simulink model "hip_controller_2026_01_27"  (R2024b)
settings: Solver=FixedStepAuto  StartTime=0.0  StopTime=simDuration  FixedStep=0.01  RelTol=1e-3  EnableMultiTasking=on
InitFcn:
  | breakp=[-1, -0.8, -0.6, -0.4, -0.2, -0.1, 0, 0.1, 0.2, 0.4, 0.6, 0.8, 1];
  | splinenew =[-1, -0.8, -0.6, -0.4, -0.2, -0.1, 0, 0, 0.005, 0.01, 0.015,0.02,0.025];
undefined symbols (not defined in the file or in its folder): Discrete, K, qbreak, Time
libraries: simulink x53, arduinolib x11, dspswit3 x9, ctrlSharedLib x2, dspfdesign x2, slpidlib x2
(part 1 of 4)
settings Model: ExtModeTrigDuration=2  Creator=Aries  LastModifiedBy=zglin
settings SolverCC: ConcurrentTasks=on  AlgebraicLoopSolver=TrustRegion  PositivePriorityOrder=on  AutoInsertRateTranBlk=on
settings DataIOCC: SaveFormat=Array  ReturnWorkspaceOutputs=off
settings OptimizationCC: ReuseModelBlockBuffer=off  PassReuseOutputArgsAs=Individual arguments  MaxStackSize=64  EfficientTunableParamExpr=on
settings DebuggingCC: ParameterTunabilityLossMsg=error  UnconnectedInputMsg=warning  UnconnectedOutputMsg=warning  UnconnectedLineMsg=warning  ArithmeticOperatorsInVariantConditions=warning
settings HardwareCC: ProdBitPerPointer=32  ProdBitPerSizeT=32  ProdBitPerPtrDiffT=32  ProdLargestAtomicInteger=Long  ProdLargestAtomicFloat=Double  ProdWordSize=32  ProdHWDeviceType=ARM Compatible->ARM Cortex
settings ModelReferenceCC: EnableRefExpFcnMdlSchedulingChecks=on
settings SFSimCC: SimUseLocalCustomCode=off  MATLABDynamicMemAlloc=off  CustomCodeUndefinedFunction=UseInterfaceOnly
settings RTWCC: Description=Embedded Coder  SystemTargetFile=ert.tlc  HardwareBoard=Arduino MKR WiFi 1010  TemplateMakefile=ert_default_tmf  GenerateReport=on  RTWUseLocalCustomCode=off  Toolchain=Arduino ARM  BuildConfiguration=Faster Runs  LaunchReport=on  GPUComputeCapability=3.5  DLArmComputeVersion=19.05
settings CodeAppCC: ForceParamTrailComments=on  IgnoreCustomStorageClasses=off  OperatorAnnotations=on  StateflowObjectComments=on  MATLABSourceComments=on
settings ERTTargetCC: SupportContinuousTime=on  SupportNonInlinedSFcns=on  SupportVariableSizeSignals=on  ExtModeTransport=3  ExtModeStaticAlloc=on  ExtModeStaticAllocSize=8192  ExtModeMexFile=ext_xcp  ExtModeIntrfLevel=Level2 - Open  InlinedParameterPlacement=Hierarchical  DynamicArrayContainerType=coder::array
settings ConfigComp: CovMetricSettings=dswe

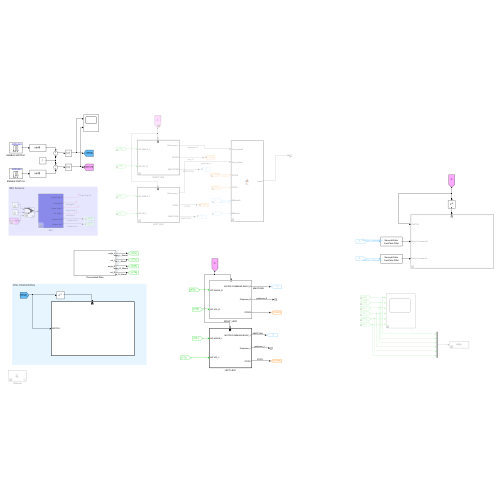
[thumbnail: Simulink's stored preview of the top-level diagram]
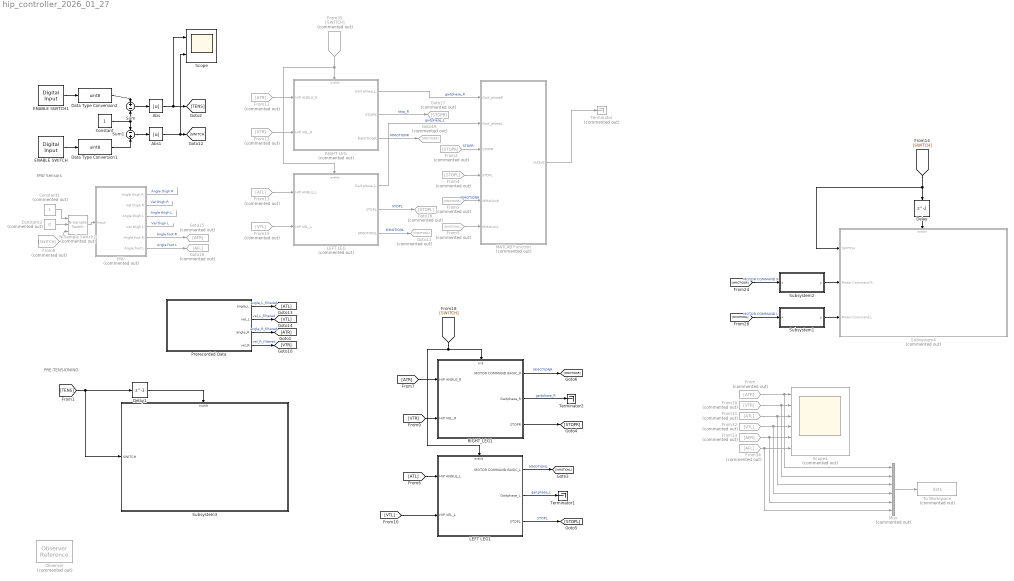
== system hip_controller_2026_01_27 ==
  note: IMU Sensors
  note: PRE-TENSIONING
  Abs : Abs  SaturateOnIntegerOverflow=off
  Abs1 : Abs  SaturateOnIntegerOverflow=off
  Constant : Constant
  Constant1 : Constant  Commented=on
  Constant3 : Constant  Commented=on  Value=0
  Data Type Conversion1 : DataTypeConversion  OutDataTypeStr=uint8  SaturateOnIntegerOverflow=off  RndMeth=Floor
  Data Type Conversion2 : DataTypeConversion  OutDataTypeStr=uint8  SaturateOnIntegerOverflow=off  RndMeth=Floor
  Delay : Delay
  Delay1 : Delay  DelayLength=1
  ENABLE SWITCH : arduinolib/Digital Input  pinNumber=6  mode=Input Pullup  Direction=input  SampleTime=0.01  blockPlatform=arduino
      settings: SourceProductName=Common
  ENABLE SWITCH1 : arduinolib/Digital Input  pinNumber=4  mode=Input Pullup  Direction=input  SampleTime=0.01  blockPlatform=arduino
      settings: SourceProductName=Common
  From : From  Commented=on  GotoTag=ATR
  From11 : From  Commented=on  GotoTag=ATR
  From12 : From  Commented=on  GotoTag=VTR
  From13 : From  Commented=on  GotoTag=ATL
  From15 : From  Commented=on  GotoTag=VTL
  From2 : From  Commented=on  GotoTag=STOPR
  From3 : From  Commented=on  GotoTag=MMOTIONR
  From30 : From  Commented=on  GotoTag=VTR
  From31 : From  Commented=on  GotoTag=ATL
  From32 : From  Commented=on  GotoTag=VTL
  From33 : From  Commented=on  GotoTag=AFR
  From34 : From  Commented=on  GotoTag=AFL
  From35 : From  Commented=on  GotoTag=SWITCH
  From4 : From  Commented=on  GotoTag=STOPL
  From5 : From  Commented=on  GotoTag=MMOTIONL
  From8 : From  Commented=on  GotoTag=SWITCH
  Goto11 : Goto  Commented=on  GotoTag=MMOTIONL
  Goto15 : Goto  Commented=on  GotoTag=AFR
  Goto16 : Goto  Commented=on  GotoTag=AFL
  Goto17 : Goto  Commented=on  GotoTag=STOPR
  Goto18 : Goto  Commented=on  GotoTag=STOPL
  Goto19 : Goto  Commented=on  GotoTag=MMOTIONR
  IMU : Subsystem  Commented=on
  LEFT LEG : Subsystem  Commented=on
  LEFT LEG1 : Subsystem
  MATLAB Function : MATLAB Function  Commented=on  TreatAsAtomicUnit=on
  Mux : Mux  Commented=on  Inputs=6
  N-Sample Switch2 : dspswit3/N-Sample Switch  Commented=on  N=10  reset=on  TriggerType=Rising edge  Ts=-1
  Observer : ObserverReference  Commented=on  ObserverModelName=hip_controller_181225_Observer1
  Prerecorded Data : Subsystem
  RIGHT LEG : Subsystem  Commented=on
  RIGHT_LEG1 : Subsystem
      settings: PortSchema="{\"entries\":[{\"content\":{\"sides\":[{\"content\":{\"connectorIds\":[\"In1\",\"In2\"]},\"type\":\"ConnectorPlacement.EquallySpacedRectSide\",\"uuid\":\"3c7f0152-c48a-47e5-a5d6-06ce9a094da4\"},{\"content\":{\"connectorIds\":[\"Out1\",\"Out2\",\"Out3\"],\"side\":\"RIGHT\"},\"type\":\"ConnectorPlacement.EquallySpacedRectSide\",\"uuid\":\"7e131d28-dc3d-49bf-b06d-5233735629db\"},{\"content\":{\"connectorIds\":[\"In3\"],\"side\":\"TOP\"},\"type\":\"ConnectorPlacement.EquallySpacedRectSide\",\"uuid\":\"34b65df0-5bb0-4402-bac3-467a5037582a\"}]},\"type\":\"ConnectorPlacement.EquallySpacedConnector\",\"uuid\":\"f00ff79e-fc41-40e3-bf13-a356f406cdad\"}],\"packageUris\":[\"http://schema.mathworks.com/mf0/Connector/R2020b\"],\"version\":\"1.0\"}"
  Scope : Scope  NumInputPorts=2
  Scope1 : Scope  Commented=on  NumInputPorts=6
  Subsystem1 : Subsystem  mask{wn=60, zt=1, x0=0}
      mask prompts: wn "Cut-off frequency (rad/s)"; zt "Damping ratio"; x0 "Initial Condition"
      mask Display: disp('Second-Order\nLow-Pass Filter');
  Subsystem2 : Subsystem  mask{wn=60, zt=1, x0=0}
      mask prompts: wn "Cut-off frequency (rad/s)"; zt "Damping ratio"; x0 "Initial Condition"
      mask Display: disp('Second-Order\nLow-Pass Filter');
  Subsystem3 : Subsystem
  Subsystem4 : Subsystem  Commented=on
  Sum : Sum  Inputs=+-
  Sum1 : Sum  Inputs=-+
  Terminator : Terminator  Commented=on
  Terminator1 : Terminator
  Terminator2 : Terminator
  To Workspace : ToWorkspace  Commented=on  VariableName=data  SampleTime=-1
      settings: Save2DSignal=2-D array (concatenate along first dimension)
  wires:
  [SWITCH] -> Delay/1, Subsystem4/1(SWITCH)
  Delay/1 -> Subsystem4/Enable
  From31/1 -> Scope1/3, Mux/3
  Constant3/1 -> N-Sample Switch2/2
  [MMOTIONL] -> Subsystem1/1(x)  "MOTOR COMMAND L"
  From34/1 -> Scope1/6, Mux/6
  From8/1 -> N-Sample Switch2/3
  From33/1 -> Scope1/5, Mux/5
  [MMOTIONR] -> Subsystem2/1(x)  "MOTOR COMMAND R"
  LEFT LEG/3(MMOTIONL) -> Goto11/1  "MMOTIONL"
  Constant1/1 -> N-Sample Switch2/1
  IMU/6(Angle foot L) -> Goto16/1  "Angle foot L"
  From13/1 -> LEFT LEG/1(HIP ANGLE_L)
  RIGHT LEG/2(STOPR) -> Goto17/1  "stop_R"
  Mux/1 -> To Workspace/1
  From12/1 -> RIGHT LEG/2(HIP VEL_R)
  N-Sample Switch2/1 -> IMU/1(Input)
  ENABLE SWITCH/1 -> Data Type Conversion1/1
  From35/1 -> RIGHT LEG/Enable, LEFT LEG/Enable
  Data Type Conversion1/1 -> Sum1/2
  RIGHT LEG/3(MMOTIONR) -> Goto19/1  "MMOTIONR"
  From11/1 -> RIGHT LEG/1(HIP ANGLE_R)
  IMU/1(Angle thigh R) -> ?  "Angle thigh R"
  From30/1 -> Mux/2, Scope1/2
  IMU/2(Vel thigh R) -> ?  "Vel thigh R"
  From32/1 -> Scope1/4, Mux/4
  IMU/5(Angle foot R) -> Goto15/1  "Angle foot R"
  From/1 -> Mux/1, Scope1/1
  IMU/4(Vel thigh L) -> ?  "Vel thigh L"
  IMU/3(Angle thigh L) -> ?  "Angle thigh L"
  LEFT LEG/2(STOPL) -> Goto18/1  "STOPL"
  From15/1 -> LEFT LEG/2(HIP VEL_L)
  Subsystem2/1(y) -> Subsystem4/2(Motor Command R)
  Subsystem1/1(y) -> Subsystem4/3(Motor Command L)
  ENABLE SWITCH1/1 -> Data Type Conversion2/1
  Data Type Conversion2/1 -> Sum/1
  Constant/1 -> Sum/2, Sum1/1
  Sum1/1 -> Abs1/1
  Sum/1 -> Abs/1
  Abs/1 -> Scope/1, [TENS]
  Abs1/1 -> Scope/2, [SWITCH]
  Delay1/1 -> Subsystem3/Enable
  [TENS] -> Subsystem3/1(SWITCH), Delay1/1
  RIGHT LEG/1(Gait phase_L) -> MATLAB Function/1(Gait_phaseR)  "gaitphase_R"
  LEFT LEG/1(Gait phase_L) -> MATLAB Function/2(Gait_phaseL)  "gaitphase_L"
  Prerecorded Data/1(angle_L) -> [ATL]  "angle_L_filtered"
  Prerecorded Data/2(vel_L) -> [VTL]  "vel_L_filtered"
  Prerecorded Data/3(angle_R) -> [ATR]  "angle_R_filtered"
  Prerecorded Data/4(vel_R) -> [VTR]  "vel_R_filtered"
  From2/1 -> MATLAB Function/3(STOPR)  "STOPR"
  From3/1 -> MATLAB Function/5(MMotionR)  "MMOTIONR"
  From4/1 -> MATLAB Function/4(STOPL)
  From5/1 -> MATLAB Function/6(MMotionL)
  MATLAB Function/1(output) -> Terminator/1
  RIGHT_LEG1/1(MOTOR COMMAND BASIC_R) -> [MMOTIONR]  "MMOTIONR"
  [VTL] -> LEFT LEG1/2(HIP VEL_L)
  [ATL] -> LEFT LEG1/1(HIP ANGLE_L)
  LEFT LEG1/3(STOPL) -> [STOPL]  "STOPL"
  [VTR] -> RIGHT_LEG1/2(HIP VEL_R)
  [SWITCH] -> RIGHT_LEG1/3(In3), LEFT LEG1/Enable
  LEFT LEG1/2(Gaitphase_L) -> Terminator1/1  "gaitphase_L"
  [ATR] -> RIGHT_LEG1/1(HIP ANGLE_R)
  LEFT LEG1/1(MOTOR COMMAND BASIC_L) -> [MMOTIONL]  "MMOTIONL"
  RIGHT_LEG1/3(STOPR) -> [STOPR]
  RIGHT_LEG1/2(Gaitphase_R) -> Terminator2/1  "gaitphase_R"

== system hip_controller_2026_01_27/IMU ==
  Input : Inport
  Data Type Conversion2 : DataTypeConversion  OutDataTypeStr=double  SaturateOnIntegerOverflow=off  RndMeth=Floor
  Demux : Demux  Outputs=6
  Gain{,2,4..5} (4 alike) : Gain  Gain=-pi/180
  Gain1 : Gain  Gain=pi/180
  Gain3 : Gain  Gain=pi/180
  IMUs (2 Thighs + 2 Feet) : arduinolib/I2C Read  I2CModule=0  Mode=Master  SlaveAddress=45  SlaveByteOrder=LittleEndian  Direction=Receiver  RegisterAddressMode=off  RegisterAddress=0  SlaveDataType=single  DataLength=6  NoAck=off  RepeatedStart=off  OutputStatus=off  blockPlatform=ARDUINO  SampleTime=0.01
      settings: SourceProductName=Common
  Remove offset : Subsystem
  Sum : Sum  Inputs=+-
  Angle thigh R : Outport
  Vel thigh R : Outport  Port=2
  Angle thigh L : Outport  Port=3
  Vel thigh L : Outport  Port=4
  Angle foot R : Outport  Port=5
  Angle foot L : Outport  Port=6
  wires:
  IMUs (2 Thighs + 2 Feet)/1 -> Data Type Conversion2/1
  Demux/5 -> Gain4/1  "Angle foot R"
  Demux/4 -> Gain3/1  "Vel thigh L"
  Demux/3 -> Gain/1  "Angle thigh L"
  Demux/2 -> Gain2/1  "Vel thigh R"
  Demux/1 -> Gain1/1  "Angle thigh R"
  Demux/6 -> Gain5/1  "Angle foot L"
  Input/1 -> Remove offset/Enable
  Data Type Conversion2/1 -> Sum/1, Remove offset/1(Input)
  Sum/1 -> Demux/1
  Remove offset/1(Mean value) -> Sum/2
  Gain/1 -> Angle thigh L/1
  Gain1/1 -> Angle thigh R/1
  Gain2/1 -> Vel thigh R/1
  Gain3/1 -> Vel thigh L/1
  Gain4/1 -> Angle foot R/1
  Gain5/1 -> Angle foot L/1

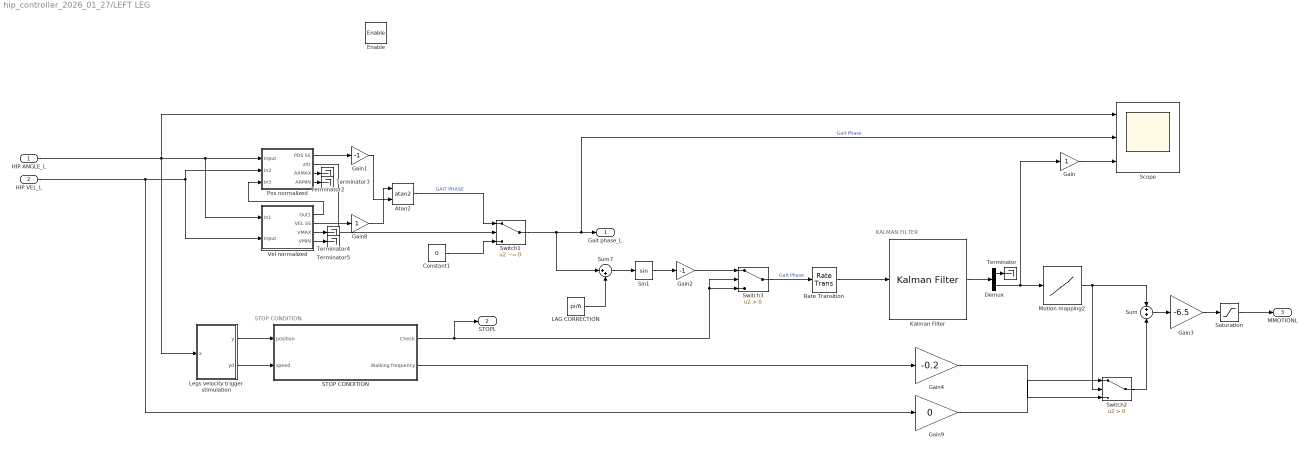
== system hip_controller_2026_01_27/LEFT LEG ==
  note: STOP CONDITION
  note: KALMAN FILTER
  HIP ANGLE_L : Inport
  HIP VEL_L : Inport  Port=2
  Enable : EnablePort  StatesWhenEnabling=reset
  Atan2 : Trigonometry  Operator=atan2
  Constant1 : Constant  Value=0
  Demux : Demux  Outputs=2
  Gain : Gain
  Gain1 : Gain  Gain=-1
  Gain2 : Gain  Gain=-1
  Gain3 : Gain  Gain=-6.5
  Gain4 : Gain  Gain=-0.2
  Gain8 : Gain
  Gain9 : Gain  Gain=0
  Kalman Filter : ctrlSharedLib/Kalman Filter  TimeDomain=Discrete-Time  UseCurrentEstimator=on  ModelSource=Individual A, B, C, D matrices  ModelSourceVariable=idss  A=[1 0.01;0 1]  B=eye(2)  C=[1 0]  D=zeros(2)  NumberOfStates=1  NumberOfInputs=1  NumberOfOutputs=1  InitialEstimateSource=Dialog  X0=0  P0=10  UseK=off  UseGH=off  NumberOfProcessNoiseInputs=2  G=1  TimeInvariantG=on  H=0  TimeInvariantH=on  Q=0.02  TimeInvariantQ=on  R=0.75  TimeInvariantR=on  N=0  TimeInvariantN=on  AddInputPort=off  AddEnablePort=off  OutputEstimatedY=off  OutputP=off  Ts=-1
  LAG CORRECTION : Constant  Value=pi/6
  Legs velocity trigger stimulation : Subsystem  mask{wn=10, zt=1, x0=0}
      mask prompts: wn "Cut-off frequency (rad/s)"; zt "Damping ratio"; x0 "Initial Condition"
      mask Display: disp('Second-Order\nLow-Pass Filter');
  Motion mapping2 : Lookup_n-D  NumberOfTableDimensions=1  BreakpointsForDimension1=breakp  BreakpointsForDimension2=qbreak(:,2)  Table=splinenew  InterpMethod=Cubic spline  ExtrapMethod=Cubic spline  InternalRulePriority=Speed  RndMeth=Simplest
  Pos normalized : Subsystem
  Rate Transition : RateTransition  OutPortSampleTime=0.01
  STOP CONDITION : Subsystem
  Saturation : Saturate  UpperLimit=600*pi/180  LowerLimit=-600*pi/180
  Scope : Scope  NumInputPorts=3
  Sin1 : Trigonometry
  Sum : Sum
  Sum7 : Sum  Inputs=|++
  Switch1 : Switch  Criteria=u2 ~= 0  SaturateOnIntegerOverflow=off  InputSameDT=off
  Switch2 : Switch  Criteria=u2 > Threshold  SaturateOnIntegerOverflow=off  InputSameDT=off
  Switch3 : Switch  Criteria=u2 > Threshold  SaturateOnIntegerOverflow=off  InputSameDT=off
  Terminator{,2..5} (5 alike) : Terminator
  Vel normalized : Subsystem
  Gait phase_L : Outport
  STOPL : Outport  Port=2
  MMOTIONL : Outport  Port=3
  wires:
  Kalman Filter/1 -> Demux/1
  Gain8/1 -> Atan2/1
  Gain2/1 -> Switch3/1
  STOP CONDITION/1(Check) -> STOPL/1, Switch3/2, Switch3/3
  Gain3/1 -> Saturation/1
  Rate Transition/1 -> Kalman Filter/1
  Atan2/1 -> Switch1/1  "GAIT PHASE"
  Sin1/1 -> Gain2/1
  Switch1/1 -> Sum7/1, Scope/2, Gait phase_L/1  "Gait Phase"
  HIP VEL_L/1 -> Vel normalized/2(Input), Pos normalized/2(In2), Gain9/1
  Switch3/1 -> Rate Transition/1  "Gait Phase"
  Constant1/1 -> Switch1/3
  Motion mapping2/1 -> Sum/1, Switch2/2
  Sum/1 -> Gain3/1
  Demux/1 -> Terminator/1
  LAG CORRECTION/1 -> Sum7/2
  Sum7/1 -> Sin1/1
  Demux/2 -> Gain/1, Motion mapping2/1
  Gain1/1 -> Atan2/2
  Gain9/1 -> Switch2/1
  Gain4/1 -> Switch2/3
  Switch2/1 -> Sum/2
  STOP CONDITION/2(Walking frequency) -> Gain4/1
  Saturation/1 -> MMOTIONL/1
  HIP ANGLE_L/1 -> Legs velocity trigger stimulation/1(x), Scope/1, Vel normalized/1(In1), Pos normalized/1(Input)
  Pos normalized/1(POS SS) -> Gain1/1
  Pos normalized/2(z(t)) -> Switch1/2
  Vel normalized/1(Out1) -> Pos normalized/3(In3)
  Vel normalized/2(VEL SS) -> Gain8/1
  Pos normalized/3(ARMAX) -> Terminator2/1
  Pos normalized/4(ARMIN) -> Terminator3/1
  Vel normalized/3(VMAX) -> Terminator4/1
  Vel normalized/4(VMIN) -> Terminator5/1
  Gain/1 -> Scope/3
  Legs velocity trigger stimulation/1(y) -> STOP CONDITION/1(position)
  Legs velocity trigger stimulation/2(yd) -> STOP CONDITION/2(speed)

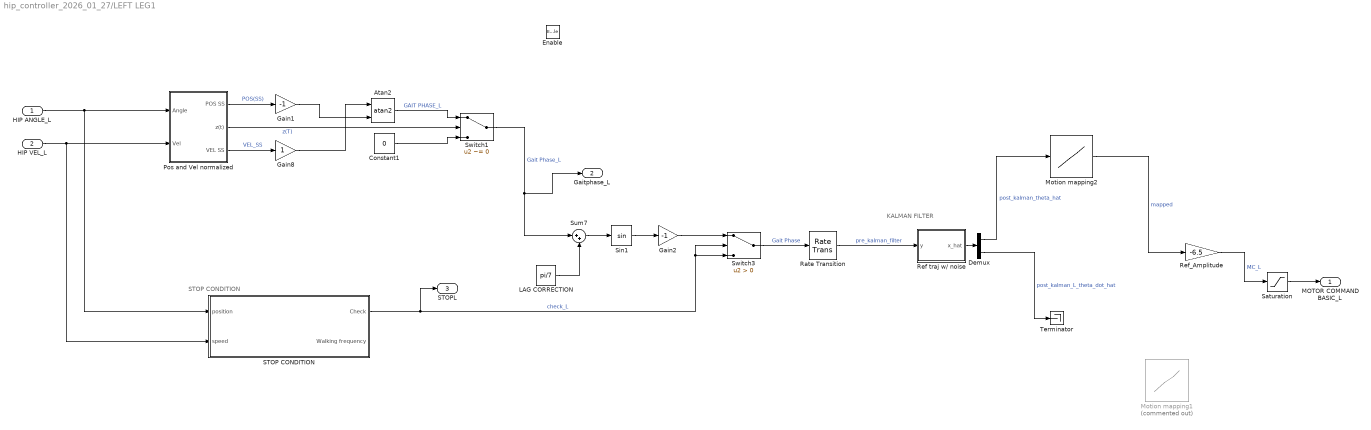
== system hip_controller_2026_01_27/LEFT LEG1 ==
  note: STOP CONDITION
  note: KALMAN FILTER
  HIP ANGLE_L : Inport
  HIP VEL_L : Inport  Port=2
  Enable : EnablePort
  Atan2 : Trigonometry  Operator=atan2
  Constant1 : Constant  Value=0
  Demux : Demux  Outputs=2
  Gain1 : Gain  Gain=-1
  Gain2 : Gain  Gain=-1
  Gain8 : Gain
  LAG CORRECTION : Constant  Value=pi/7
  Motion mapping1 : Lookup_n-D  Commented=on  NumberOfTableDimensions=1  BreakpointsForDimension1=[-1, -0.8, -0.6, -0.4, -0.2, -0.1, 0, 0.1, 0.2, 0.4, 0.6, 0.8, 1]  BreakpointsForDimension2=qbreak(:,2)  Table=[-1, -0.8, -0.6, -0.4, -0.2, -0.1, 0, 0, 0.005, 0.01, 0.015,0.02,0.025]  InterpMethod=Cubic spline  ExtrapMethod=Cubic spline  InternalRulePriority=Speed  RndMeth=Simplest
  Motion mapping2 : Lookup_n-D  NumberOfTableDimensions=1  BreakpointsForDimension1=breakp  BreakpointsForDimension2=qbreak(:,2)  Table=splinenew  InterpMethod=Cubic spline  ExtrapMethod=Cubic spline  InternalRulePriority=Speed  RndMeth=Simplest
  Pos and Vel normalized : Subsystem
  Rate Transition : RateTransition  OutPortSampleTime=0.01
  Ref traj w/ noise : MATLAB Function  TreatAsAtomicUnit=on
  Ref_Amplitude : Gain  Gain=-6.5
  STOP CONDITION : Subsystem
  Saturation : Saturate  UpperLimit=600*pi/180  LowerLimit=-600*pi/180
  Sin1 : Trigonometry
  Sum7 : Sum  Inputs=|++
  Switch1 : Switch  Criteria=u2 ~= 0  SaturateOnIntegerOverflow=off  InputSameDT=off
  Switch3 : Switch  Criteria=u2 > Threshold  SaturateOnIntegerOverflow=off  InputSameDT=off
  Terminator : Terminator
  MOTOR COMMAND BASIC_L : Outport
  Gaitphase_L : Outport  Port=2
  STOPL : Outport  Port=3
  wires:
  Gain8/1 -> Atan2/1
  Gain2/1 -> Switch3/1
  STOP CONDITION/1(Check) -> STOPL/1, Switch3/2, Switch3/3  "check_L"
  Atan2/1 -> Switch1/1  "GAIT PHASE_L"
  Sin1/1 -> Gain2/1
  Switch1/1 -> Sum7/1, Gaitphase_L/1  "Gait Phase_L"
  Switch3/1 -> Rate Transition/1  "Gait Phase"
  Constant1/1 -> Switch1/3
  LAG CORRECTION/1 -> Sum7/2
  Sum7/1 -> Sin1/1
  Gain1/1 -> Atan2/2
  Pos and Vel normalized/1(POS SS) -> Gain1/1  "POS(SS)"
  Pos and Vel normalized/2(z(t)) -> Switch1/2  "z(T)"
  Pos and Vel normalized/3(VEL SS) -> Gain8/1  "VEL_SS"
  Demux/1 -> Motion mapping2/1  "post_kalman_theta_hat"
  Motion mapping2/1 -> Ref_Amplitude/1  "mapped"
  Ref_Amplitude/1 -> Saturation/1  "MC_L"
  HIP VEL_L/1 -> Pos and Vel normalized/2(Vel), STOP CONDITION/2(speed)
  HIP ANGLE_L/1 -> Pos and Vel normalized/1(Angle), STOP CONDITION/1(position)
  Rate Transition/1 -> Ref traj w/ noise/1(y)  "pre_kalman_filter"
  Ref traj w/ noise/1(x_hat) -> Demux/1
  Demux/2 -> Terminator/1  "post_kalman_L_theta_dot_hat"
  Saturation/1 -> MOTOR COMMAND BASIC_L/1

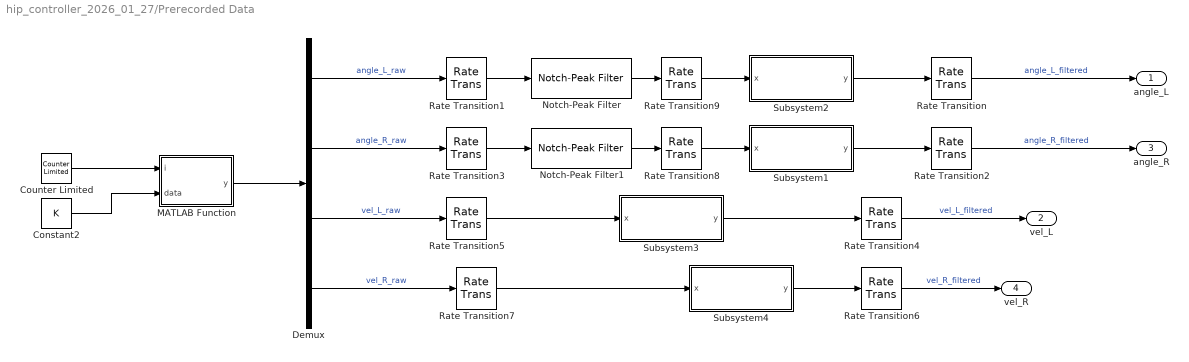
== system hip_controller_2026_01_27/Prerecorded Data ==
  Constant2 : Constant  Value=K
  Counter Limited : simulink/Sources/Counter Limited  uplimit=size(K,1)  tsamp=0.01
  Demux : Demux
  MATLAB Function : MATLAB Function  TreatAsAtomicUnit=on
  Notch-Peak Filter : dspfdesign/Notch-Peak Filter  Specification=Bandwidth and center frequency  BandwidthPort=off  Bandwidth=0.1  QualityFactorPort=off  QualityFactor=5  CenterFrequencyPort=off  CenterFrequency=0  BandwidthCoefficientPort=off  BandwidthCoefficient=0.72654  CenterFrequencyCoefficientPort=off  CenterFrequencyCoefficient=0  Output=Notch  SampleRateMode=Specify on dialog  SampleRate=100  SimulateUsing=Interpreted execution
  Notch-Peak Filter1 : dspfdesign/Notch-Peak Filter  Specification=Bandwidth and center frequency  BandwidthPort=off  Bandwidth=0.1  QualityFactorPort=off  QualityFactor=5  CenterFrequencyPort=off  CenterFrequency=0  BandwidthCoefficientPort=off  BandwidthCoefficient=0.72654  CenterFrequencyCoefficientPort=off  CenterFrequencyCoefficient=0  Output=Notch  SampleRateMode=Specify on dialog  SampleRate=100  SimulateUsing=Interpreted execution
  Rate Transition{,1..9} (10 alike) : RateTransition  OutPortSampleTime=0.01
  Subsystem1 : Subsystem  mask{wn=20, zt=1, x0=0}
      mask prompts: wn "Cut-off frequency (rad/s)"; zt "Damping ratio"; x0 "Initial Condition"
      mask Display: disp('Second-Order\nLow-Pass Filter');
  Subsystem2 : Subsystem  mask{wn=20, zt=1, x0=0}
      mask prompts: wn "Cut-off frequency (rad/s)"; zt "Damping ratio"; x0 "Initial Condition"
      mask Display: disp('Second-Order\nLow-Pass Filter');
  Subsystem3 : Subsystem  mask{wn=20, zt=1, x0=0}
      mask prompts: wn "Cut-off frequency (rad/s)"; zt "Damping ratio"; x0 "Initial Condition"
      mask Display: disp('Second-Order\nLow-Pass Filter');
  Subsystem4 : Subsystem  mask{wn=20, zt=1, x0=0}
      mask prompts: wn "Cut-off frequency (rad/s)"; zt "Damping ratio"; x0 "Initial Condition"
      mask Display: disp('Second-Order\nLow-Pass Filter');
  angle_L : Outport
  vel_L : Outport  Port=2
  angle_R : Outport  Port=3
  vel_R : Outport  Port=4
  wires:
  Notch-Peak Filter/1 -> Rate Transition9/1
  Rate Transition1/1 -> Notch-Peak Filter/1
  Rate Transition3/1 -> Notch-Peak Filter1/1
  MATLAB Function/1(y) -> Demux/1
  Counter Limited/1 -> MATLAB Function/1(i)
  Constant2/1 -> MATLAB Function/2(data)
  Notch-Peak Filter1/1 -> Rate Transition8/1
  Demux/1 -> Rate Transition1/1  "angle_L_raw"
  Demux/2 -> Rate Transition3/1  "angle_R_raw"
  Rate Transition2/1 -> angle_R/1  "angle_R_filtered"
  Rate Transition/1 -> angle_L/1  "angle_L_filtered"
  Subsystem2/1(y) -> Rate Transition/1
  Subsystem1/1(y) -> Rate Transition2/1
  Subsystem3/1(y) -> Rate Transition4/1
  Rate Transition5/1 -> Subsystem3/1(x)
  Rate Transition4/1 -> vel_L/1  "vel_L_filtered"
  Demux/3 -> Rate Transition5/1  "vel_L_raw"
  Rate Transition7/1 -> Subsystem4/1(x)
  Subsystem4/1(y) -> Rate Transition6/1
  Demux/4 -> Rate Transition7/1  "vel_R_raw"
  Rate Transition6/1 -> vel_R/1  "vel_R_filtered"
  Rate Transition9/1 -> Subsystem2/1(x)
  Rate Transition8/1 -> Subsystem1/1(x)

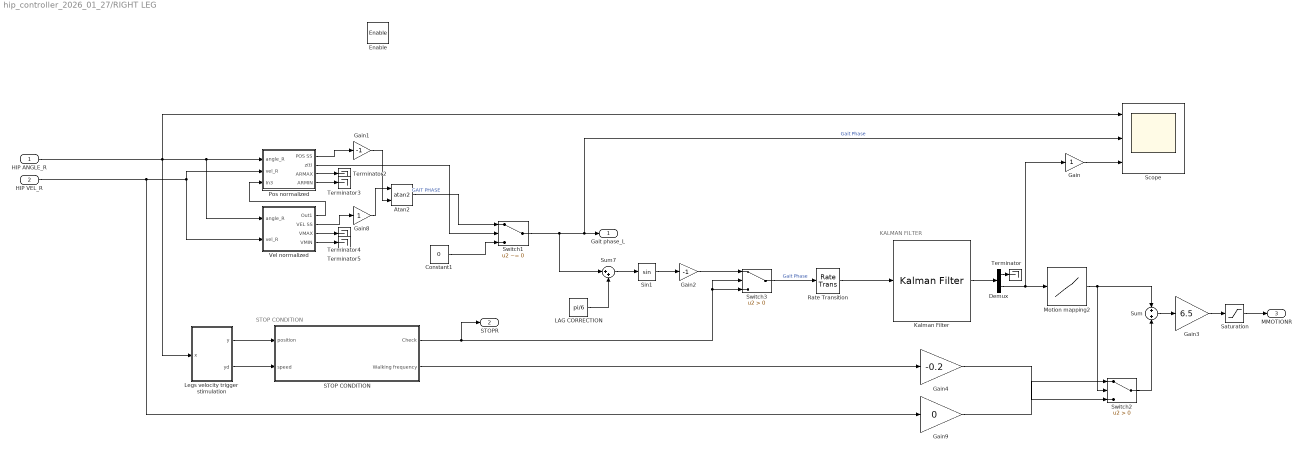
== system hip_controller_2026_01_27/RIGHT LEG ==
  note: STOP CONDITION
  note: KALMAN FILTER
  HIP ANGLE_R : Inport
  HIP VEL_R : Inport  Port=2
  Enable : EnablePort  StatesWhenEnabling=reset
  Atan2 : Trigonometry  Operator=atan2
  Constant1 : Constant  Value=0
  Demux : Demux  Outputs=2
  Gain : Gain
  Gain1 : Gain  Gain=-1
  Gain2 : Gain  Gain=-1
  Gain3 : Gain  Gain=6.5
  Gain4 : Gain  Gain=-0.2
  Gain8 : Gain
  Gain9 : Gain  Gain=0
  Kalman Filter : ctrlSharedLib/Kalman Filter  TimeDomain=Discrete-Time  UseCurrentEstimator=on  ModelSource=Individual A, B, C, D matrices  ModelSourceVariable=idss  A=[1 0.01;0 1]  B=eye(2)  C=[1 0]  D=zeros(2)  NumberOfStates=1  NumberOfInputs=1  NumberOfOutputs=1  InitialEstimateSource=Dialog  X0=0  P0=10  UseK=off  UseGH=off  NumberOfProcessNoiseInputs=2  G=1  TimeInvariantG=on  H=0  TimeInvariantH=on  Q=0.02  TimeInvariantQ=on  R=0.75  TimeInvariantR=on  N=0  TimeInvariantN=on  AddInputPort=off  AddEnablePort=off  OutputEstimatedY=off  OutputP=off  Ts=-1
  LAG CORRECTION : Constant  Value=pi/6
  Legs velocity trigger stimulation : Subsystem  mask{wn=10, zt=1, x0=0}
      mask prompts: wn "Cut-off frequency (rad/s)"; zt "Damping ratio"; x0 "Initial Condition"
      mask Display: disp('Second-Order\nLow-Pass Filter');
  Motion mapping2 : Lookup_n-D  NumberOfTableDimensions=1  BreakpointsForDimension1=breakp  BreakpointsForDimension2=qbreak(:,2)  Table=splinenew  InterpMethod=Cubic spline  ExtrapMethod=Cubic spline  InternalRulePriority=Speed  RndMeth=Simplest
  Pos normalized : Subsystem
  Rate Transition : RateTransition  OutPortSampleTime=0.01
  STOP CONDITION : Subsystem
  Saturation : Saturate  UpperLimit=600*pi/180  LowerLimit=-600*pi/180
  Scope : Scope  NumInputPorts=3
  Sin1 : Trigonometry
  Sum : Sum
  Sum7 : Sum  Inputs=|++
  Switch1 : Switch  Criteria=u2 ~= 0  SaturateOnIntegerOverflow=off  InputSameDT=off
  Switch2 : Switch  Criteria=u2 > Threshold  SaturateOnIntegerOverflow=off  InputSameDT=off
  Switch3 : Switch  Criteria=u2 > Threshold  SaturateOnIntegerOverflow=off  InputSameDT=off
  Terminator{,2..5} (5 alike) : Terminator
  Vel normalized : Subsystem
  Gait phase_L : Outport
  STOPR : Outport  Port=2
  MMOTIONR : Outport  Port=3
  wires:
  Kalman Filter/1 -> Demux/1
  Gain8/1 -> Atan2/1
  Gain2/1 -> Switch3/1
  STOP CONDITION/1(Check) -> STOPR/1, Switch3/2, Switch3/3
  Gain3/1 -> Saturation/1
  Rate Transition/1 -> Kalman Filter/1
  Atan2/1 -> Switch1/1  "GAIT PHASE"
  Sin1/1 -> Gain2/1
  Switch1/1 -> Sum7/1, Scope/2, Gait phase_L/1  "Gait Phase"
  HIP VEL_R/1 -> Vel normalized/2(vel_R), Pos normalized/2(vel_R), Gain9/1
  Switch3/1 -> Rate Transition/1  "Gait Phase"
  Constant1/1 -> Switch1/3
  Motion mapping2/1 -> Sum/1, Switch2/2
  Sum/1 -> Gain3/1
  Demux/1 -> Terminator/1
  LAG CORRECTION/1 -> Sum7/2
  Sum7/1 -> Sin1/1
  Demux/2 -> Gain/1, Motion mapping2/1
  Gain1/1 -> Atan2/2
  Gain9/1 -> Switch2/1
  Gain4/1 -> Switch2/3
  Switch2/1 -> Sum/2
  STOP CONDITION/2(Walking frequency) -> Gain4/1
  HIP ANGLE_R/1 -> Legs velocity trigger stimulation/1(x), Scope/1, Vel normalized/1(angle_R), Pos normalized/1(angle_R)
  Pos normalized/1(POS SS) -> Gain1/1
  Pos normalized/2(z(t)) -> Switch1/2
  Vel normalized/1(Out1) -> Pos normalized/3(In3)
  Vel normalized/2(VEL SS) -> Gain8/1
  Pos normalized/3(ARMAX) -> Terminator2/1
  Pos normalized/4(ARMIN) -> Terminator3/1
  Vel normalized/3(VMAX) -> Terminator4/1
  Vel normalized/4(VMIN) -> Terminator5/1
  Gain/1 -> Scope/3
  Legs velocity trigger stimulation/1(y) -> STOP CONDITION/1(position)
  Legs velocity trigger stimulation/2(yd) -> STOP CONDITION/2(speed)
  Saturation/1 -> MMOTIONR/1

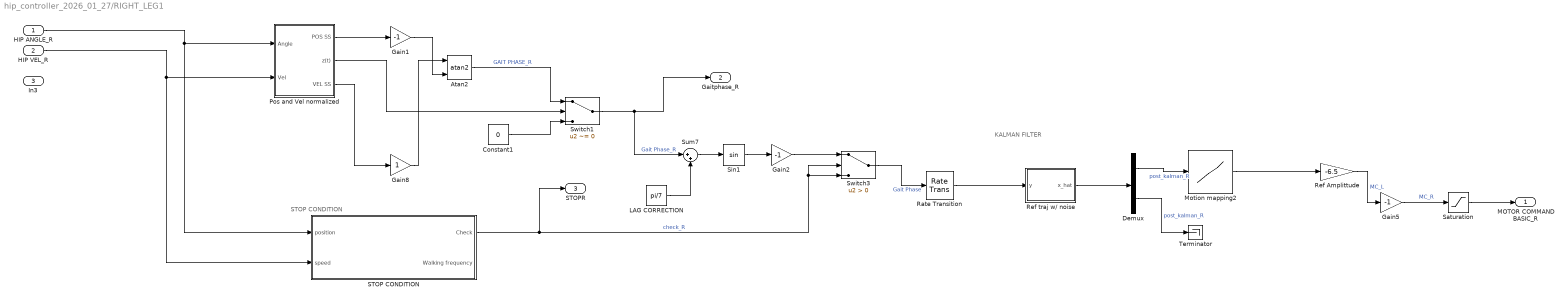
== system hip_controller_2026_01_27/RIGHT_LEG1 ==
  note: STOP CONDITION
  note: KALMAN FILTER
  HIP ANGLE_R : Inport
  HIP VEL_R : Inport  Port=2
  In3 : Inport  Port=3
  Atan2 : Trigonometry  Operator=atan2
  Constant1 : Constant  Value=0
  Demux : Demux  Outputs=2
  Gain1 : Gain  Gain=-1
  Gain2 : Gain  Gain=-1
  Gain5 : Gain  Gain=-1
  Gain8 : Gain
  LAG CORRECTION : Constant  Value=pi/7
  Motion mapping2 : Lookup_n-D  NumberOfTableDimensions=1  BreakpointsForDimension1=breakp  BreakpointsForDimension2=qbreak(:,2)  Table=splinenew  InterpMethod=Cubic spline  ExtrapMethod=Cubic spline  InternalRulePriority=Speed  RndMeth=Simplest
  Pos and Vel normalized : Subsystem
  Rate Transition : RateTransition  OutPortSampleTime=0.01
  Ref Amplittude : Gain  Gain=-6.5
  Ref traj w/ noise : MATLAB Function  TreatAsAtomicUnit=on
  STOP CONDITION : Subsystem
  Saturation : Saturate  UpperLimit=600*pi/180  LowerLimit=-600*pi/180
  Sin1 : Trigonometry
  Sum7 : Sum  Inputs=|++
  Switch1 : Switch  Criteria=u2 ~= 0  SaturateOnIntegerOverflow=off  InputSameDT=off
  Switch3 : Switch  Criteria=u2 > Threshold  SaturateOnIntegerOverflow=off  InputSameDT=off
  Terminator : Terminator
  MOTOR COMMAND BASIC_R : Outport
  Gaitphase_R : Outport  Port=2
  STOPR : Outport  Port=3
  wires:
  Gain8/1 -> Atan2/1
  Gain2/1 -> Switch3/1
  STOP CONDITION/1(Check) -> STOPR/1, Switch3/2, Switch3/3  "check_R"
  Atan2/1 -> Switch1/1  "GAIT PHASE_R"
  Sin1/1 -> Gain2/1
  Switch1/1 -> Sum7/1, Gaitphase_R/1  "Gait Phase_R"
  HIP VEL_R/1 -> Pos and Vel normalized/2(Vel), STOP CONDITION/2(speed)
  Switch3/1 -> Rate Transition/1  "Gait Phase"
  Constant1/1 -> Switch1/3
  LAG CORRECTION/1 -> Sum7/2
  Sum7/1 -> Sin1/1
  Gain1/1 -> Atan2/2
  Pos and Vel normalized/1(POS SS) -> Gain1/1
  Pos and Vel normalized/2(z(t)) -> Switch1/2
  Pos and Vel normalized/3(VEL SS) -> Gain8/1
  HIP ANGLE_R/1 -> STOP CONDITION/1(position), Pos and Vel normalized/1(Angle)
  Demux/1 -> Motion mapping2/1  "post_kalman_R"
  Motion mapping2/1 -> Ref Amplittude/1
  Gain5/1 -> Saturation/1  "MC_R"
  Ref Amplittude/1 -> Gain5/1  "MC_L"
  Rate Transition/1 -> Ref traj w/ noise/1(y)
  Ref traj w/ noise/1(x_hat) -> Demux/1
  Saturation/1 -> MOTOR COMMAND BASIC_R/1
  Demux/2 -> Terminator/1  "post_kalman_R"

== system hip_controller_2026_01_27/Subsystem1 ==
  x : Inport
  Constant : Constant  Value=2
  Integrator1 : Integrator  InitialConditionSource=external
  Integrator2 : Integrator
  Product : Product  RndMeth=Zero
  Product1 : Product  RndMeth=Zero
  Product2 : Product  Inputs=3  RndMeth=Zero
  Sum : Sum  Inputs=|+-
  Sum1 : Sum  Inputs=|+-
  wn : Constant  Value=wn
  x0 : Constant  Value=x0
  zt : Constant  Value=zt
  y : Outport  VectorParamsAs1DForOutWhenUnconnected=off
  wires:
  Sum/1 -> Product/2
  wn/1 -> Product/1, Product1/1
  Sum1/1 -> Sum/1
  x0/1 -> Integrator1/2
  Integrator2/1 -> Product1/2, Product2/1
  Product/1 -> Integrator2/1
  x/1 -> Sum1/1
  Product1/1 -> Integrator1/1
  Integrator1/1 -> Sum1/2, y/1
  Product2/1 -> Sum/2
  zt/1 -> Product2/3
  Constant/1 -> Product2/2

== system hip_controller_2026_01_27/Subsystem2 ==
  x : Inport
  Constant : Constant  Value=2
  Integrator1 : Integrator  InitialConditionSource=external
  Integrator2 : Integrator
  Product : Product  RndMeth=Zero
  Product1 : Product  RndMeth=Zero
  Product2 : Product  Inputs=3  RndMeth=Zero
  Sum : Sum  Inputs=|+-
  Sum1 : Sum  Inputs=|+-
  wn : Constant  Value=wn
  x0 : Constant  Value=x0
  zt : Constant  Value=zt
  y : Outport  VectorParamsAs1DForOutWhenUnconnected=off
  wires:
  Sum/1 -> Product/2
  wn/1 -> Product/1, Product1/1
  Sum1/1 -> Sum/1
  x0/1 -> Integrator1/2
  Integrator2/1 -> Product1/2, Product2/1
  Product/1 -> Integrator2/1
  x/1 -> Sum1/1
  Product1/1 -> Integrator1/1
  Integrator1/1 -> Sum1/2, y/1
  Product2/1 -> Sum/2
  zt/1 -> Product2/3
  Constant/1 -> Product2/2

== system hip_controller_2026_01_27/Subsystem3 ==
  note: RightLeg_AK60-6 Motor Modules
  note: LeftLeg_AK60-6 Motor Modules
  SWITCH : Inport
  Enable : EnablePort  StatesWhenEnabling=reset
  Abs : Abs  SaturateOnIntegerOverflow=off
  Abs1 : Abs  SaturateOnIntegerOverflow=off
  Chart : Stateflow chart  TreatAsAtomicUnit=on
  Chart1 : Stateflow chart  TreatAsAtomicUnit=on
  Data Type Conversion1 : DataTypeConversion  OutDataTypeStr=single  SaturateOnIntegerOverflow=off  RndMeth=Floor
  Data Type Conversion6 : DataTypeConversion  OutDataTypeStr=single  SaturateOnIntegerOverflow=off  RndMeth=Floor
  Left Motor Velocity : Subsystem
  Right Motor Velocity : Subsystem
  Subsystem1 : Subsystem  mask{wn=25, zt=1, x0=0}
      mask prompts: wn "Cut-off frequency (rad/s)"; zt "Damping ratio"; x0 "Initial Condition"
      mask Display: disp('Second-Order\nLow-Pass Filter');
  Subsystem4 : Subsystem  mask{wn=25, zt=1, x0=0}
      mask prompts: wn "Cut-off frequency (rad/s)"; zt "Damping ratio"; x0 "Initial Condition"
      mask Display: disp('Second-Order\nLow-Pass Filter');
  Terminator{1..6} (6 alike) : Terminator
  wires:
  Chart1/2(vel) -> Data Type Conversion1/1
  SWITCH/1 -> Chart1/2(ON_OFF), Chart/2(ON_OFF)
  Data Type Conversion6/1 -> Right Motor Velocity/2(Motor command)
  Left Motor Velocity/3(MOTOR TORQUE) -> Subsystem1/1(x)
  Right Motor Velocity/2(MOTOR SPEED) -> Terminator2/1
  Left Motor Velocity/2(MOTOR SPEED) -> Terminator1/1
  Chart/2(vel) -> Data Type Conversion6/1
  Right Motor Velocity/1(MOTOR POSITION) -> Terminator4/1
  Subsystem4/1(y) -> Abs/1  "TORQUE"
  Right Motor Velocity/3(MOTOR TORQUE) -> Subsystem4/1(x)
  Subsystem4/2(yd) -> Terminator5/1
  Abs/1 -> Chart/1(MOTOR_TORQUE)
  Left Motor Velocity/1(MOTOR POSITION) -> Terminator3/1
  Subsystem1/1(y) -> Abs1/1  "TORQUE"
  Subsystem1/2(yd) -> Terminator6/1
  Abs1/1 -> Chart1/1(MOTOR_TORQUE)
  Chart/1(enablestati) -> Right Motor Velocity/1(SWITCH)
  Chart1/1(enablestati) -> Left Motor Velocity/1(SWITCH)
  Data Type Conversion1/1 -> Left Motor Velocity/2(Motor command)

== system hip_controller_2026_01_27/Subsystem4 ==
  note: RightLeg_AK60-6 Motor Modules
  note: LeftLeg_AK60-6 Motor Modules
  SWITCH : Inport
  Motor Command R : Inport  Port=2
  Motor Command L : Inport  Port=3
  Enable : EnablePort  StatesWhenEnabling=reset
  Data Type Conversion3 : DataTypeConversion  OutDataTypeStr=single  SaturateOnIntegerOverflow=off  RndMeth=Floor
  Data Type Conversion6 : DataTypeConversion  OutDataTypeStr=single  SaturateOnIntegerOverflow=off  RndMeth=Floor
  Left Motor Velocity : Subsystem
  PID1 : Subsystem  Commented=on
  PID2 : Subsystem  Commented=on
  PID3 : Subsystem
  PID4 : Subsystem
  Right Motor Velocity : Subsystem
  Terminator{1..3,14} (4 alike) : Terminator
  wires:
  Data Type Conversion3/1 -> Left Motor Velocity/2(Motor command)
  Right Motor Velocity/1(MOTOR POSITION) -> PID3/2(Actual Motion)
  PID3/1(Velocity output) -> Data Type Conversion6/1
  Right Motor Velocity/3(MOTOR TORQUE) -> Terminator3/1
  SWITCH/1 -> PID4/Enable, Left Motor Velocity/1(SWITCH), PID3/Enable, Right Motor Velocity/1(SWITCH)
  Motor Command R/1 -> PID3/1(Ref)
  Data Type Conversion6/1 -> Right Motor Velocity/2(Motor command)
  PID4/1(Velocity output) -> Data Type Conversion3/1
  Left Motor Velocity/3(MOTOR TORQUE) -> Terminator14/1
  Left Motor Velocity/1(MOTOR POSITION) -> PID4/2(Actual Motion)
  Right Motor Velocity/2(MOTOR SPEED) -> Terminator2/1
  Left Motor Velocity/2(MOTOR SPEED) -> Terminator1/1
  Motor Command L/1 -> PID4/1(Ref)

== system hip_controller_2026_01_27/IMU/Remove offset ==
  Input : Inport
  Enable : EnablePort  StatesWhenEnabling=reset
  Constant1 : Constant
  Divide : Product  Inputs=*/
  Memory : Memory
  Memory1 : Memory
  Sum of Elements : Sum
  Sum of Elements1 : Sum
  Mean value : Outport
  wires:
  Input/1 -> Sum of Elements/2
  Sum of Elements/1 -> Divide/1, Memory/1  "Sum of elements"
  Memory/1 -> Sum of Elements/1
  Memory1/1 -> Sum of Elements1/1
  Sum of Elements1/1 -> Divide/2, Memory1/1  "Counter"
  Constant1/1 -> Sum of Elements1/2
  Divide/1 -> Mean value/1

== system hip_controller_2026_01_27/LEFT LEG/Legs velocity trigger stimulation ==
  x : Inport
  Constant : Constant  Value=2
  Integrator1 : Integrator  InitialConditionSource=external
  Integrator2 : Integrator
  Product : Product  RndMeth=Zero
  Product1 : Product  RndMeth=Zero
  Product2 : Product  Inputs=3  RndMeth=Zero
  Sum : Sum  Inputs=|+-
  Sum1 : Sum  Inputs=|+-
  wn : Constant  Value=wn
  x0 : Constant  Value=x0
  zt : Constant  Value=zt
  y : Outport  VectorParamsAs1DForOutWhenUnconnected=off
  yd : Outport  Port=2  VectorParamsAs1DForOutWhenUnconnected=off
  wires:
  Sum/1 -> Product/2
  wn/1 -> Product/1, Product1/1
  Sum1/1 -> Sum/1
  x0/1 -> Integrator1/2
  Integrator2/1 -> Product1/2, Product2/1
  Product/1 -> Integrator2/1
  x/1 -> Sum1/1
  Product1/1 -> Integrator1/1, yd/1
  Integrator1/1 -> Sum1/2, y/1
  Product2/1 -> Sum/2
  zt/1 -> Product2/3
  Constant/1 -> Product2/2

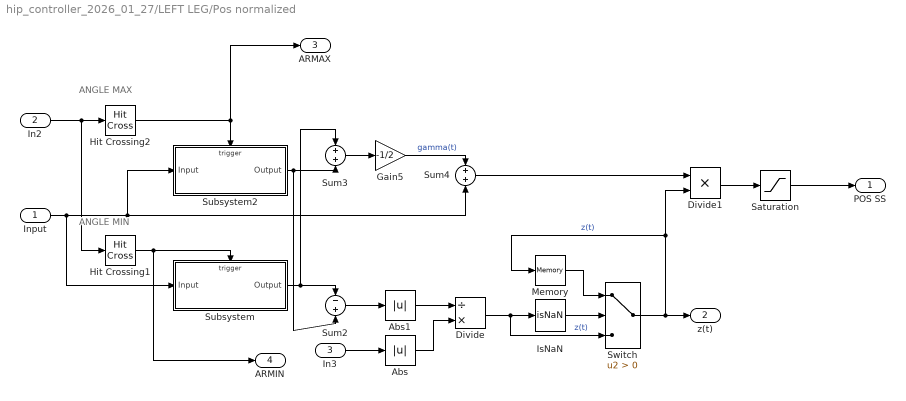
== system hip_controller_2026_01_27/LEFT LEG/Pos normalized ==
  note: ANGLE MIN
  note: ANGLE MAX
  Input : Inport
  In2 : Inport  Port=2
  In3 : Inport  Port=3
  Abs : Abs  SaturateOnIntegerOverflow=off
  Abs1 : Abs  SaturateOnIntegerOverflow=off
  Divide : Product  Inputs=/*
  Divide1 : Product  Inputs=**
  Gain5 : Gain  Gain=-1/2
  Hit Crossing1 : HitCross  HitCrossingOffset=-1  HitCrossingDirection=rising
  Hit Crossing2 : HitCross  HitCrossingOffset=1  HitCrossingDirection=falling
  IsNaN : RelationalOperator  Operator=isNaN  OutDataTypeStr=boolean  RndMeth=Simplest  InputSameDT=off
  Memory : Memory
  Saturation : Saturate  UpperLimit=10  LowerLimit=-10
  Subsystem : Subsystem
  Subsystem2 : Subsystem
  Sum2 : Sum  Inputs=-+
  Sum3 : Sum
  Sum4 : Sum
  Switch : Switch  Criteria=u2 > Threshold  SaturateOnIntegerOverflow=off  InputSameDT=off
  POS SS : Outport
  z(t) : Outport  Port=2
  ARMAX : Outport  Port=3
  ARMIN : Outport  Port=4
  wires:
  Hit Crossing2/1 -> Subsystem2/Trigger, ARMAX/1
  Subsystem2/1(Output) -> Sum3/2, Sum2/2
  Sum4/1 -> Divide1/1
  Sum3/1 -> Gain5/1
  Subsystem/1(Output) -> Sum2/1, Sum3/1
  Hit Crossing1/1 -> ARMIN/1, Subsystem/Trigger
  Input/1 -> Subsystem2/1(Input), Sum4/2, Subsystem/1(Input)
  In2/1 -> Hit Crossing1/1, Hit Crossing2/1
  Sum2/1 -> Abs1/1
  In3/1 -> Abs/1
  Gain5/1 -> Sum4/1  "gamma(t)"
  Abs1/1 -> Divide/1
  Abs/1 -> Divide/2
  Divide/1 -> IsNaN/1, Switch/3  "z(t)"
  Memory/1 -> Switch/1
  IsNaN/1 -> Switch/2
  Switch/1 -> Memory/1, Divide1/2, z(t)/1  "z(t)"
  Divide1/1 -> Saturation/1
  Saturation/1 -> POS SS/1

== system hip_controller_2026_01_27/LEFT LEG/STOP CONDITION ==
  position : Inport
  speed : Inport  Port=2
  Constant : Constant
  Constant1 : Constant  Value=0
  Sqrt : Sqrt
  Square : Math  Operator=square
  Square1 : Math  Operator=square
  Sum : Sum
  Switch3 : Switch  Criteria=u2 > Threshold  Threshold=0.3  SaturateOnIntegerOverflow=off  InputSameDT=off
  Check : Outport
  Walking frequency : Outport  Port=2
  wires:
  position/1 -> Square/1  "θ"
  speed/1 -> Square1/1  "θ_dot"
  Square/1 -> Sum/1
  Square1/1 -> Sum/2
  Sum/1 -> Sqrt/1
  Constant/1 -> Switch3/1
  Constant1/1 -> Switch3/3
  Sqrt/1 -> Switch3/2, Walking frequency/1
  Switch3/1 -> Check/1

== system hip_controller_2026_01_27/LEFT LEG/Vel normalized ==
  note: SPEED MAX
  note: SPEED MIN
  In1 : Inport
  Input : Inport  Port=2
  Gain7 : Gain  Gain=-1/2
  Hit Crossing3 : HitCross  HitCrossingOffset=-0.1  HitCrossingDirection=rising
  Hit Crossing4 : HitCross  HitCrossingOffset=0.1  HitCrossingDirection=falling
  Subsystem1 : Subsystem
  Subsystem3 : Subsystem
  Sum1 : Sum  Inputs=+-
  Sum5 : Sum
  Sum6 : Sum
  Out1 : Outport
  VEL SS : Outport  Port=2
  VMAX : Outport  Port=3
  VMIN : Outport  Port=4
  wires:
  Sum5/1 -> Gain7/1
  Subsystem1/1(Output) -> Sum1/1, Sum5/1
  Sum1/1 -> Out1/1
  Subsystem3/1(Output) -> Sum1/2, Sum5/2
  In1/1 -> Hit Crossing4/1, Hit Crossing3/1
  Gain7/1 -> Sum6/2  "GAMMA(t)"
  Sum6/1 -> VEL SS/1
  Input/1 -> Sum6/1, Subsystem1/1(Input), Subsystem3/1(Input)
  Hit Crossing3/1 -> VMIN/1, Subsystem1/Trigger
  Hit Crossing4/1 -> VMAX/1, Subsystem3/Trigger

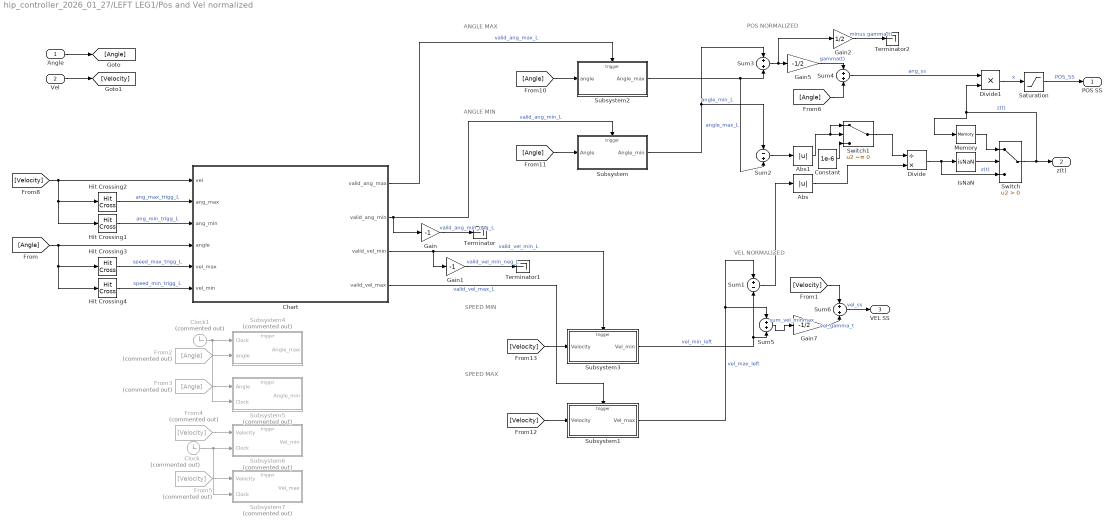
== system hip_controller_2026_01_27/LEFT LEG1/Pos and Vel normalized ==
  note: ANGLE MIN
  note: ANGLE MAX
  note: SPEED MAX
  note: SPEED MIN
  note: POS NORMALIZED
  note: VEL NORMALIZED
  Angle : Inport
  Vel : Inport  Port=2
  Abs : Abs  SaturateOnIntegerOverflow=off
  Abs1 : Abs  SaturateOnIntegerOverflow=off
  Chart : Stateflow chart  TreatAsAtomicUnit=on
      settings: PortSchema="{\"entries\":[{\"content\":{\"sides\":[{\"content\":{\"connectorIds\":[\"In5\",\"In1\",\"In4\",\"In6\",\"In3\",\"In2\"]},\"type\":\"ConnectorPlacement.EquallySpacedRectSide\",\"uuid\":\"1b4e9464-0c1b-4aef-9691-eb83c0a92a72\"},{\"content\":{\"connectorIds\":[\"Out3\",\"Out4\",\"Out2\",\"Out1\"],\"side\":\"RIGHT\"},\"type\":\"ConnectorPlacement.EquallySpacedRectSide\",\"uuid\":\"791196f6-4c97-40a1-8015-a03f83b94293\"},{\"content\":{\"side\":\"TOP\"},\"type\":\"ConnectorPlacement.EquallySpacedRectSide\",\"uuid\":\"116d3fb6-be2c-4be4-86cc-df9779b501c6\"}]},\"type\":\"ConnectorPlacement.EquallySpacedConnector\",\"uuid\":\"13d090b2-a2d1-429a-b321-7320a6f027c7\"}],\"packageUris\":[\"http://schema.mathworks.com/mf0/Connector/R2020b\"],\"version\":\"1.0\"}"
  Clock : Clock  Commented=on
  Clock1 : Clock  Commented=on
  Constant : Constant  Value=1e-6
  Divide : Product  Inputs=/*
  Divide1 : Product  Inputs=**
  From2 : From  Commented=on  GotoTag=Angle
  From3 : From  Commented=on  GotoTag=Angle
  From4 : From  Commented=on  GotoTag=Velocity
  From5 : From  Commented=on  GotoTag=Velocity
  Gain : Gain  Gain=-1
  Gain1 : Gain  Gain=-1
  Gain2 : Gain  Gain=1/2
  Gain5 : Gain  Gain=-1/2
  Gain7 : Gain  Gain=-1/2
  Hit Crossing1 : HitCross  HitCrossingDirection=rising
  Hit Crossing2 : HitCross  HitCrossingDirection=falling
  Hit Crossing3 : HitCross  HitCrossingDirection=rising
  Hit Crossing4 : HitCross  HitCrossingDirection=falling
  IsNaN : RelationalOperator  Operator=isNaN  OutDataTypeStr=boolean  RndMeth=Simplest  InputSameDT=off
  Memory : Memory
  Saturation : Saturate  UpperLimit=10  LowerLimit=-10
  Subsystem : Subsystem
  Subsystem1 : Subsystem
  Subsystem2 : Subsystem
  Subsystem3 : Subsystem
  Subsystem4 : Subsystem  Commented=on
  Subsystem5 : Subsystem  Commented=on
  Subsystem6 : Subsystem  Commented=on
  Subsystem7 : Subsystem  Commented=on
  Sum1 : Sum  Inputs=+-
  Sum2 : Sum  Inputs=-+
  Sum{3..6} (4 alike) : Sum
  Switch : Switch  Criteria=u2 > Threshold  SaturateOnIntegerOverflow=off  InputSameDT=off
  Switch1 : Switch  Criteria=u2 ~= 0  SaturateOnIntegerOverflow=off  InputSameDT=off
  Terminator : Terminator
  Terminator1 : Terminator
  Terminator2 : Terminator
  POS SS : Outport
  z(t) : Outport  Port=2
  VEL SS : Outport  Port=3
  wires:
  Hit Crossing2/1 -> Chart/1(ang_max)  "ang_max_trigg_L"
  Subsystem2/1(Angle_max) -> Sum2/2, Sum3/2  "angle_max_L"
  Sum4/1 -> Divide1/1  "ang_ss"
  Sum3/1 -> Gain2/1, Gain5/1
  Subsystem/1(Angle_min) -> Sum2/1, Sum3/1  "angle_min_L"
  Hit Crossing1/1 -> Chart/4(ang_min)  "ang_min_trigg_L"
  Sum2/1 -> Abs1/1
  Sum1/1 -> Abs/1
  Gain5/1 -> Sum4/1  "gamma(t)"
  Abs/1 -> Divide/2
  Divide/1 -> IsNaN/1, Switch/3  "z(t)"
  Memory/1 -> Switch/1
  IsNaN/1 -> Switch/2
  Switch/1 -> Memory/1, Divide1/2, z(t)/1  "z(t)"
  Divide1/1 -> Saturation/1  "x"
  Saturation/1 -> POS SS/1  "POS_SS"
  Clock1/1 -> Subsystem5/2(Clock), Subsystem4/1(Clock)
  Constant/1 -> Switch1/3
  Abs1/1 -> Switch1/2, Switch1/1
  Switch1/1 -> Divide/1
  Clock/1 -> Subsystem7/2(Clock), Subsystem6/2(Clock)
  Hit Crossing4/1 -> Chart/2(vel_min)  "speed_min_trigg_L"
  Subsystem3/1(Vel_min) -> Sum1/2, Sum5/2  "vel_min_left"
  Subsystem1/1(Vel_max) -> Sum1/1, Sum5/1  "vel_max_left"
  Sum5/1 -> Gain7/1  "sum_vel_minmax"
  Hit Crossing3/1 -> Chart/3(vel_max)  "speed_max_trigg_L"
  Sum6/1 -> VEL SS/1  "vel_ss"
  Gain7/1 -> Sum6/2  "vel_gamma_t"
  [Velocity] -> Sum6/1
  Chart/1(valid_vel_max) -> Subsystem1/Trigger  "valid_vel_max_L"
  Chart/4(valid_ang_min) -> Gain/1, Subsystem/Trigger  "valid_ang_min_L"
  Chart/3(valid_ang_max) -> Subsystem2/Trigger  "valid_ang_max_L"
  Chart/2(valid_vel_min) -> Gain1/1, Subsystem3/Trigger  "valid_vel_min_L"
  Vel/1 -> [Velocity]
  Angle/1 -> [Angle]
  From5/1 -> Subsystem7/1(Velocity)
  From4/1 -> Subsystem6/1(Velocity)
  From3/1 -> Subsystem5/1(Angle)
  From2/1 -> Subsystem4/2(angle)
  [Angle] -> Hit Crossing4/1, Hit Crossing3/1, Chart/6(angle)
  [Angle] -> Subsystem/1(Angle)
  [Angle] -> Subsystem2/1(angle)
  [Velocity] -> Subsystem1/1(Velocity)
  [Velocity] -> Subsystem3/1(Velocity)
  [Velocity] -> Hit Crossing1/1, Hit Crossing2/1, Chart/5(vel)
  Gain/1 -> Terminator/1  "valid_ang_min_neg_L"
  Gain1/1 -> Terminator1/1  "valid_vel_min_neg_L"
  [Angle] -> Sum4/2
  Gain2/1 -> Terminator2/1  "minus gamma(t)"

== system hip_controller_2026_01_27/LEFT LEG1/STOP CONDITION ==
  position : Inport
  speed : Inport  Port=2
  Constant : Constant
  Constant1 : Constant  Value=0
  Sqrt : Sqrt
  Square : Math  Operator=square
  Square1 : Math  Operator=square
  Sum : Sum
  Switch3 : Switch  Criteria=u2 > Threshold  Threshold=0.3  SaturateOnIntegerOverflow=off  InputSameDT=off
  Check : Outport
  Walking frequency : Outport  Port=2
  wires:
  position/1 -> Square/1  "θ"
  speed/1 -> Square1/1  "θ_dot"
  Square/1 -> Sum/1
  Square1/1 -> Sum/2
  Sum/1 -> Sqrt/1
  Constant/1 -> Switch3/1
  Constant1/1 -> Switch3/3
  Sqrt/1 -> Switch3/2, Walking frequency/1
  Switch3/1 -> Check/1

== system hip_controller_2026_01_27/Prerecorded Data/Subsystem1 ==
  x : Inport
  Constant : Constant  Value=2
  Integrator1 : Integrator  InitialConditionSource=external
  Integrator2 : Integrator
  Product : Product  RndMeth=Zero
  Product1 : Product  RndMeth=Zero
  Product2 : Product  Inputs=3  RndMeth=Zero
  Sum : Sum  Inputs=|+-
  Sum1 : Sum  Inputs=|+-
  wn : Constant  Value=wn
  x0 : Constant  Value=x0
  zt : Constant  Value=zt
  y : Outport  VectorParamsAs1DForOutWhenUnconnected=off
  wires:
  Sum/1 -> Product/2
  wn/1 -> Product/1, Product1/1
  Sum1/1 -> Sum/1
  x0/1 -> Integrator1/2
  Integrator2/1 -> Product1/2, Product2/1
  Product/1 -> Integrator2/1
  x/1 -> Sum1/1
  Product1/1 -> Integrator1/1
  Integrator1/1 -> Sum1/2, y/1
  Product2/1 -> Sum/2
  zt/1 -> Product2/3
  Constant/1 -> Product2/2

== system hip_controller_2026_01_27/Prerecorded Data/Subsystem2 ==
  x : Inport
  Constant : Constant  Value=2
  Integrator1 : Integrator  InitialConditionSource=external
  Integrator2 : Integrator
  Product : Product  RndMeth=Zero
  Product1 : Product  RndMeth=Zero
  Product2 : Product  Inputs=3  RndMeth=Zero
  Sum : Sum  Inputs=|+-
  Sum1 : Sum  Inputs=|+-
  wn : Constant  Value=wn
  x0 : Constant  Value=x0
  zt : Constant  Value=zt
  y : Outport  VectorParamsAs1DForOutWhenUnconnected=off
  wires:
  Sum/1 -> Product/2
  wn/1 -> Product/1, Product1/1
  Sum1/1 -> Sum/1
  x0/1 -> Integrator1/2
  Integrator2/1 -> Product1/2, Product2/1
  Product/1 -> Integrator2/1
  x/1 -> Sum1/1
  Product1/1 -> Integrator1/1
  Integrator1/1 -> Sum1/2, y/1
  Product2/1 -> Sum/2
  zt/1 -> Product2/3
  Constant/1 -> Product2/2

== system hip_controller_2026_01_27/Prerecorded Data/Subsystem3 ==
  x : Inport
  Constant : Constant  Value=2
  Integrator1 : Integrator  InitialConditionSource=external
  Integrator2 : Integrator
  Product : Product  RndMeth=Zero
  Product1 : Product  RndMeth=Zero
  Product2 : Product  Inputs=3  RndMeth=Zero
  Sum : Sum  Inputs=|+-
  Sum1 : Sum  Inputs=|+-
  wn : Constant  Value=wn
  x0 : Constant  Value=x0
  zt : Constant  Value=zt
  y : Outport  VectorParamsAs1DForOutWhenUnconnected=off
  wires:
  Sum/1 -> Product/2
  wn/1 -> Product/1, Product1/1
  Sum1/1 -> Sum/1
  x0/1 -> Integrator1/2
  Integrator2/1 -> Product1/2, Product2/1
  Product/1 -> Integrator2/1
  x/1 -> Sum1/1
  Product1/1 -> Integrator1/1
  Integrator1/1 -> Sum1/2, y/1
  Product2/1 -> Sum/2
  zt/1 -> Product2/3
  Constant/1 -> Product2/2

== system hip_controller_2026_01_27/Prerecorded Data/Subsystem4 ==
  x : Inport
  Constant : Constant  Value=2
  Integrator1 : Integrator  InitialConditionSource=external
  Integrator2 : Integrator
  Product : Product  RndMeth=Zero
  Product1 : Product  RndMeth=Zero
  Product2 : Product  Inputs=3  RndMeth=Zero
  Sum : Sum  Inputs=|+-
  Sum1 : Sum  Inputs=|+-
  wn : Constant  Value=wn
  x0 : Constant  Value=x0
  zt : Constant  Value=zt
  y : Outport  VectorParamsAs1DForOutWhenUnconnected=off
  wires:
  Sum/1 -> Product/2
  wn/1 -> Product/1, Product1/1
  Sum1/1 -> Sum/1
  x0/1 -> Integrator1/2
  Integrator2/1 -> Product1/2, Product2/1
  Product/1 -> Integrator2/1
  x/1 -> Sum1/1
  Product1/1 -> Integrator1/1
  Integrator1/1 -> Sum1/2, y/1
  Product2/1 -> Sum/2
  zt/1 -> Product2/3
  Constant/1 -> Product2/2

== system hip_controller_2026_01_27/RIGHT LEG/Legs velocity trigger stimulation ==
  x : Inport
  Constant : Constant  Value=2
  Integrator1 : Integrator  InitialConditionSource=external
  Integrator2 : Integrator
  Product : Product  RndMeth=Zero
  Product1 : Product  RndMeth=Zero
  Product2 : Product  Inputs=3  RndMeth=Zero
  Sum : Sum  Inputs=|+-
  Sum1 : Sum  Inputs=|+-
  wn : Constant  Value=wn
  x0 : Constant  Value=x0
  zt : Constant  Value=zt
  y : Outport  VectorParamsAs1DForOutWhenUnconnected=off
  yd : Outport  Port=2  VectorParamsAs1DForOutWhenUnconnected=off
  wires:
  Sum/1 -> Product/2
  wn/1 -> Product/1, Product1/1
  Sum1/1 -> Sum/1
  x0/1 -> Integrator1/2
  Integrator2/1 -> Product1/2, Product2/1
  Product/1 -> Integrator2/1
  x/1 -> Sum1/1
  Product1/1 -> Integrator1/1, yd/1
  Integrator1/1 -> Sum1/2, y/1
  Product2/1 -> Sum/2
  zt/1 -> Product2/3
  Constant/1 -> Product2/2

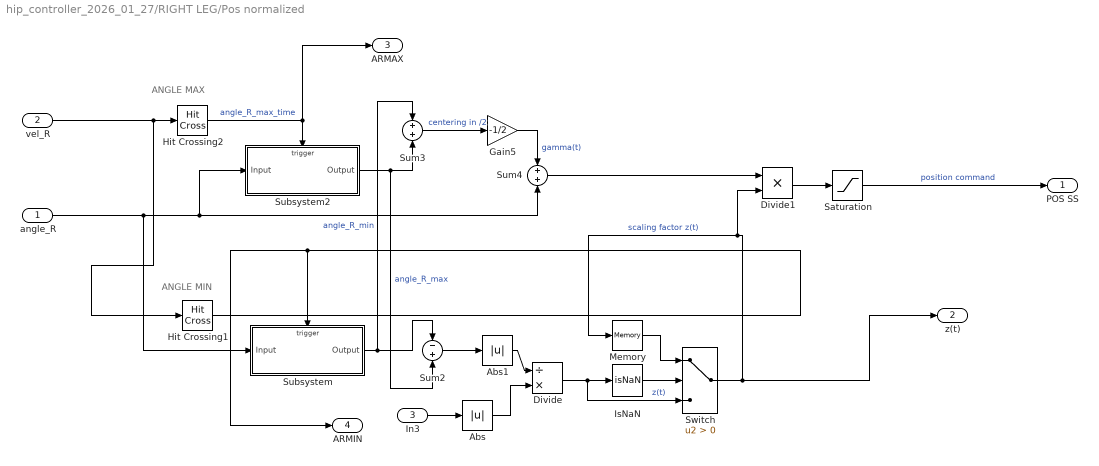
== system hip_controller_2026_01_27/RIGHT LEG/Pos normalized ==
  note: ANGLE MIN
  note: ANGLE MAX
  angle_R : Inport
  vel_R : Inport  Port=2
  In3 : Inport  Port=3
  Abs : Abs  SaturateOnIntegerOverflow=off
  Abs1 : Abs  SaturateOnIntegerOverflow=off
  Divide : Product  Inputs=/*
  Divide1 : Product  Inputs=**
  Gain5 : Gain  Gain=-1/2
  Hit Crossing1 : HitCross  HitCrossingOffset=-1  HitCrossingDirection=rising
  Hit Crossing2 : HitCross  HitCrossingOffset=1  HitCrossingDirection=falling
  IsNaN : RelationalOperator  Operator=isNaN  OutDataTypeStr=boolean  RndMeth=Simplest  InputSameDT=off
  Memory : Memory
  Saturation : Saturate  UpperLimit=10  LowerLimit=-10
  Subsystem : Subsystem
  Subsystem2 : Subsystem
  Sum2 : Sum  Inputs=-+
  Sum3 : Sum
  Sum4 : Sum
  Switch : Switch  Criteria=u2 > Threshold  SaturateOnIntegerOverflow=off  InputSameDT=off
  POS SS : Outport
  z(t) : Outport  Port=2
  ARMAX : Outport  Port=3
  ARMIN : Outport  Port=4
  wires:
  Hit Crossing2/1 -> Subsystem2/Trigger, ARMAX/1  "angle_R_max_time"
  Subsystem2/1(Output) -> Sum3/2, Sum2/2  "angle_R_max"
  Sum4/1 -> Divide1/1
  Sum3/1 -> Gain5/1  "centering in /2"
  Subsystem/1(Output) -> Sum3/1, Sum2/1  "angle_R_min"
  Hit Crossing1/1 -> ARMIN/1, Subsystem/Trigger
  angle_R/1 -> Subsystem2/1(Input), Sum4/2, Subsystem/1(Input)
  vel_R/1 -> Hit Crossing1/1, Hit Crossing2/1
  Sum2/1 -> Abs1/1
  In3/1 -> Abs/1
  Gain5/1 -> Sum4/1  "gamma(t)"
  Abs1/1 -> Divide/1
  Abs/1 -> Divide/2
  Divide/1 -> IsNaN/1, Switch/3  "z(t)"
  Memory/1 -> Switch/1
  IsNaN/1 -> Switch/2
  Switch/1 -> Memory/1, Divide1/2, z(t)/1  "scaling factor z(t)"
  Divide1/1 -> Saturation/1
  Saturation/1 -> POS SS/1  "position command"

== system hip_controller_2026_01_27/RIGHT LEG/STOP CONDITION ==
  position : Inport
  speed : Inport  Port=2
  Constant : Constant
  Constant1 : Constant  Value=0
  Sqrt : Sqrt
  Square : Math  Operator=square
  Square1 : Math  Operator=square
  Sum : Sum
  Switch3 : Switch  Criteria=u2 > Threshold  Threshold=0.3  SaturateOnIntegerOverflow=off  InputSameDT=off
  Check : Outport
  Walking frequency : Outport  Port=2
  wires:
  position/1 -> Square/1  "θ"
  speed/1 -> Square1/1  "θ_dot"
  Square/1 -> Sum/1
  Square1/1 -> Sum/2
  Sum/1 -> Sqrt/1
  Constant/1 -> Switch3/1
  Constant1/1 -> Switch3/3
  Sqrt/1 -> Switch3/2, Walking frequency/1
  Switch3/1 -> Check/1

== system hip_controller_2026_01_27/RIGHT LEG/Vel normalized ==
  note: SPEED MAX
  note: SPEED MIN
  angle_R : Inport
  vel_R : Inport  Port=2
  Gain7 : Gain  Gain=-1/2
  Hit Crossing3 : HitCross  HitCrossingOffset=-0.1  HitCrossingDirection=rising
  Hit Crossing4 : HitCross  HitCrossingOffset=0.1  HitCrossingDirection=falling
  Subsystem1 : Subsystem
  Subsystem3 : Subsystem
  Sum1 : Sum  Inputs=+-
  Sum5 : Sum
  Sum6 : Sum
  Out1 : Outport
  VEL SS : Outport  Port=2
  VMAX : Outport  Port=3
  VMIN : Outport  Port=4
  wires:
  Sum5/1 -> Gain7/1
  Subsystem1/1(Output) -> Sum1/1, Sum5/1
  Sum1/1 -> Out1/1
  Subsystem3/1(Output) -> Sum1/2, Sum5/2
  angle_R/1 -> Hit Crossing4/1, Hit Crossing3/1
  Gain7/1 -> Sum6/2  "GAMMA(t)"
  Sum6/1 -> VEL SS/1
  vel_R/1 -> Sum6/1, Subsystem1/1(Input), Subsystem3/1(Input)
  Hit Crossing3/1 -> VMIN/1, Subsystem1/Trigger
  Hit Crossing4/1 -> VMAX/1, Subsystem3/Trigger
